simulink model "Body_Dynamics"  (R2020a)
settings: Solver=ode4  StartTime=0.0  StopTime=200  FixedStep=0.01  RelTol=1e-3
values from neighbouring files (symbols this model uses):
  A =     [bluntbody_parameters.m]
  alpha = [aero_data(19:-1:1,1);aero_data(20:38,1)]    [bluntbody_parameters.m]
  Cd = [aero_data(19:-1:1,3);aero_data(20:38,3)]    [bluntbody_parameters.m]
  Cl = [aero_data(19:-1:1,2);aero_data(20:38,2)]    [bluntbody_parameters.m]
  Cmalphadot =     [bluntbody_parameters.m]
  Cmcg = [aero_data(19:-1:1,9);aero_data(20:38,9)]    [bluntbody_parameters.m]
  Cmq =     [bluntbody_parameters.m]
  D =     [bluntbody_parameters.m]
  g =     [bluntbody_parameters.m]
  Iyy =     [bluntbody_parameters.m]
  Ka =     [bluntbody_parameters.m]
  Kr =     [bluntbody_parameters.m]
  lc =     [bluntbody_parameters.m]
  LTP =     [bluntbody_parameters.m]
  m =     [bluntbody_parameters.m]
  R =     [bluntbody_parameters.m]
  RCL =     [bluntbody_parameters.m]
  Tc =     [bluntbody_parameters.m]
  UTP =     [bluntbody_parameters.m]
settings Model: Creator=nikun  LastModifiedBy=nikun

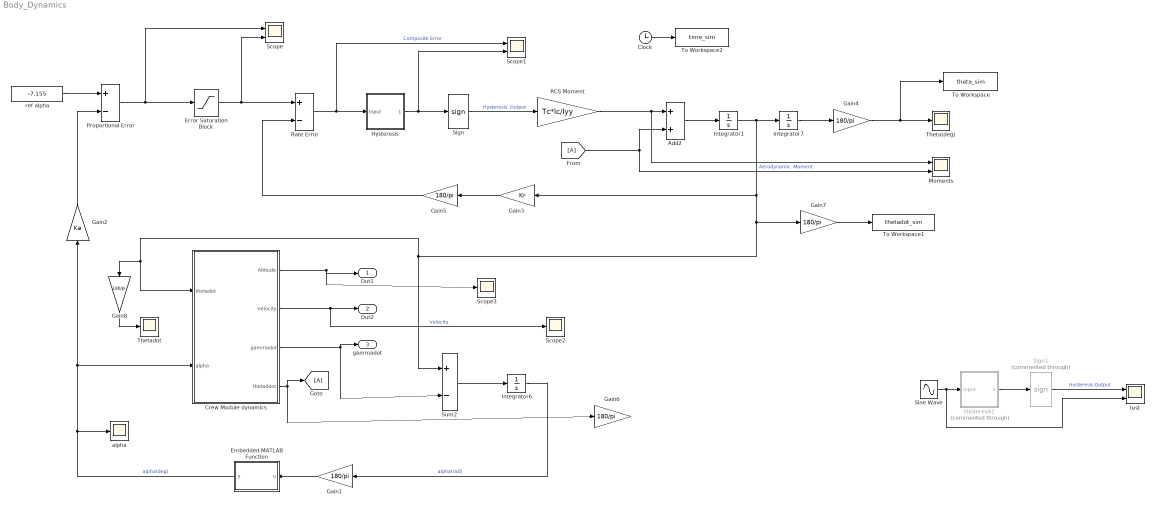
== system Body_Dynamics ==
  Add2 : Sum
  Clock : Clock
  Crew Module dynamics : Subsystem
  Embedded MATLAB Function : MATLAB Function  TreatAsAtomicUnit=on
  Error Saturation Block : Saturate  UpperLimit=RCL  LowerLimit=-RCL
  Gain{1,4..8} (6 alike) : Gain  Gain=180/pi  SaturateOnIntegerOverflow=on  OutDataTypeStr=Inherit: Same as input  ParamDataTypeStr=Inherit: Same as input
  Gain2 : Gain  Gain=Ka  SaturateOnIntegerOverflow=on  OutDataTypeStr=Inherit: Same as input  ParamDataTypeStr=Inherit: Same as input
  Gain3 : Gain  Gain=Kr  SaturateOnIntegerOverflow=on  OutDataTypeStr=Inherit: Same as input  ParamDataTypeStr=Inherit: Same as input
  Hysteresis : Subsystem
  Hysteresis1 : Subsystem  Commented=through
  Integrator1 : Integrator
  Integrator6 : Integrator  InitialCondition=150*pi/180
  Integrator7 : Integrator  InitialCondition=-2*pi/180
  Moments : Scope  NumInputPorts=2
  Proportional Error : Sum  Inputs=+-
  RCS Moment : Gain  Gain=Tc*lc/Iyy  SaturateOnIntegerOverflow=on  OutDataTypeStr=Inherit: Same as input  ParamDataTypeStr=Inherit: Same as input
  Rate Error : Sum  Inputs=+-
  Scope : Scope  NumInputPorts=2
  Scope1 : Scope  NumInputPorts=2
  Scope2 : Scope
  Scope3 : Scope
  Sign : Signum  ZeroCross=off
  Sign1 : Signum  Commented=through  ZeroCross=off
  Sine Wave : Sin  Amplitude=10  SampleTime=0
  Sum2 : Sum  Inputs=+-  InputSameDT=on  SaturateOnIntegerOverflow=on  OutDataTypeStr=Inherit: Same as first input
  Theta(deg) : Scope
  Thetadot : Scope
  To Workspace : ToWorkspace  VariableName=theta_sim  SampleTime=-1
  To Workspace1 : ToWorkspace  VariableName=thetadot_sim  SampleTime=-1
  To Workspace2 : ToWorkspace  VariableName=time_sim  SampleTime=-1
  alpha : Scope
  ref alpha : Constant  Value=-7.155
  test : Scope  NumInputPorts=2
  Out1 : Outport
  Out2 : Outport  Port=2
  gammadot : Outport  Port=3
  wires:
  Sum2/1 -> Integrator6/1
  Integrator6/1 -> Gain1/1  "alpha(rad)"
  Gain1/1 -> Embedded MATLAB Function/1(u)
  Crew Module dynamics/1(Altitude) -> Scope3/1, Out1/1
  Crew Module dynamics/2(Velocity) -> Scope2/1, Out2/1  "Velocity"
  Crew Module dynamics/3(gammadot) -> Sum2/2, gammadot/1
  Embedded MATLAB Function/1(y) -> alpha/1, Crew Module dynamics/2(alpha), Gain2/1  "alpha(deg)"
  Gain2/1 -> Proportional Error/2
  ref alpha/1 -> Proportional Error/1
  Proportional Error/1 -> Scope/1, Error Saturation Block/1
  Error Saturation Block/1 -> Scope/2, Rate Error/1
  Crew Module dynamics/4(thetaddot) -> Gain6/1, [A]
  [A] -> Moments/2, Add2/2  "Aerodynamic  Moment"
  Add2/1 -> Integrator1/1
  Integrator1/1 -> Gain3/1, Gain7/1, Gain8/1, Crew Module dynamics/1(thetadot), Sum2/1, Integrator7/1
  RCS Moment/1 -> Moments/1, Add2/1
  Sign/1 -> RCS Moment/1  "Hysteresis  Output"
  Gain3/1 -> Gain5/1
  Integrator7/1 -> Gain4/1
  Gain4/1 -> To Workspace/1, Theta(deg)/1
  Hysteresis/1(Output) -> Scope1/2, Sign/1
  Rate Error/1 -> Scope1/1, Hysteresis/1(Input)  "Composite Error"
  Gain5/1 -> Rate Error/2
  Sine Wave/1 -> test/2, Hysteresis1/1(Input)
  Hysteresis1/1(Output) -> Sign1/1
  Sign1/1 -> test/1  "Hysteresis Output"
  Gain7/1 -> To Workspace1/1
  Clock/1 -> To Workspace2/1
  Gain8/1 -> Thetadot/1

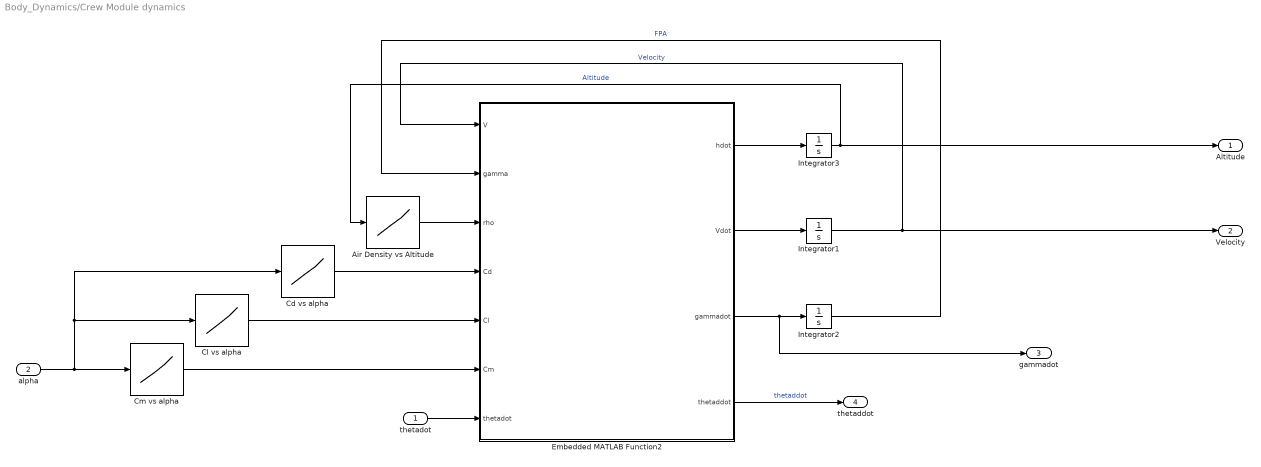
== system Body_Dynamics/Crew Module dynamics ==
  thetadot : Inport
  alpha : Inport  Port=2
  Air Density vs Altitude : Lookup_n-D  NumberOfTableDimensions=1  BreakpointsForDimension1=[0,1000,2000,3000,4000,5000,6000,7000,8000,9000,10000,12000,15000]  Table=[1.225,1.11164,1.00649,0.909122,0.819129,0.736116,0.659697,0.589501,0.525168,0.466348,0.412707,0.310828,0.193674]  InternalRulePriority=Speed  RndMeth=Simplest  InputSameDT=on
  Cd vs alpha : Lookup_n-D  NumberOfTableDimensions=1  BreakpointsForDimension1=alpha  Table=Cd  RndMeth=Simplest  InputSameDT=on
  Cl vs alpha : Lookup_n-D  NumberOfTableDimensions=1  BreakpointsForDimension1=alpha  Table=Cl  RndMeth=Simplest  InputSameDT=on
  Cm vs alpha : Lookup_n-D  NumberOfTableDimensions=1  BreakpointsForDimension1=alpha  Table=Cmcg  RndMeth=Simplest  InputSameDT=on
  Embedded MATLAB Function2 : MATLAB Function  TreatAsAtomicUnit=on
  Integrator1 : Integrator  InitialCondition=68
  Integrator2 : Integrator  InitialCondition=1*pi/180
  Integrator3 : Integrator  InitialCondition=13240
  Altitude : Outport
  Velocity : Outport  Port=2
  gammadot : Outport  Port=3
  thetaddot : Outport  Port=4
  wires:
  Embedded MATLAB Function2/4(thetaddot) -> thetaddot/1  "thetaddot"
  Embedded MATLAB Function2/2(Vdot) -> Integrator1/1
  Integrator2/1 -> Embedded MATLAB Function2/2(gamma)  "FPA"
  Integrator1/1 -> Velocity/1, Embedded MATLAB Function2/1(V)  "Velocity"
  Cl vs alpha/1 -> Embedded MATLAB Function2/5(Cl)
  alpha/1 -> Cd vs alpha/1, Cl vs alpha/1, Cm vs alpha/1
  Cd vs alpha/1 -> Embedded MATLAB Function2/4(Cd)
  Cm vs alpha/1 -> Embedded MATLAB Function2/6(Cm)
  Integrator3/1 -> Altitude/1, Air Density vs Altitude/1  "Altitude"
  Air Density vs Altitude/1 -> Embedded MATLAB Function2/3(rho)
  Embedded MATLAB Function2/1(hdot) -> Integrator3/1
  Embedded MATLAB Function2/3(gammadot) -> gammadot/1, Integrator2/1
  thetadot/1 -> Embedded MATLAB Function2/7(thetadot)

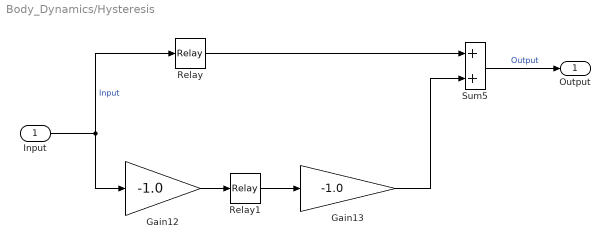
== system Body_Dynamics/Hysteresis ==
  Input : Inport
  Gain12 : Gain  Gain=-1.0  SaturateOnIntegerOverflow=on  OutDataTypeStr=Inherit: Same as input  ParamDataTypeStr=Inherit: Same as input
  Gain13 : Gain  Gain=-1.0  SaturateOnIntegerOverflow=on  OutDataTypeStr=Inherit: Same as input  ParamDataTypeStr=Inherit: Same as input
  Relay : Relay  OnSwitchValue=UTP  OffSwitchValue=LTP
  Relay1 : Relay  OnSwitchValue=UTP  OffSwitchValue=LTP
  Sum5 : Sum  InputSameDT=on  SaturateOnIntegerOverflow=on  OutDataTypeStr=Inherit: Same as first input
  Output : Outport
  wires:
  Relay/1 -> Sum5/1
  Input/1 -> Gain12/1, Relay/1  "Input"
  Sum5/1 -> Output/1  "Output"
  Gain12/1 -> Relay1/1
  Relay1/1 -> Gain13/1
  Gain13/1 -> Sum5/2

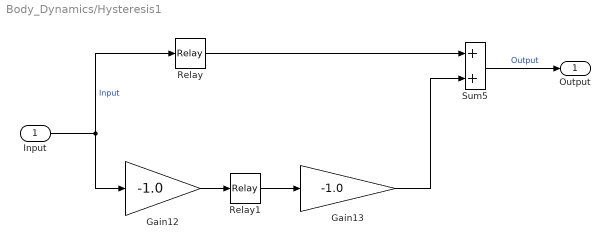
== system Body_Dynamics/Hysteresis1 ==
  Input : Inport
  Gain12 : Gain  Gain=-1.0  SaturateOnIntegerOverflow=on  OutDataTypeStr=Inherit: Same as input  ParamDataTypeStr=Inherit: Same as input
  Gain13 : Gain  Gain=-1.0  SaturateOnIntegerOverflow=on  OutDataTypeStr=Inherit: Same as input  ParamDataTypeStr=Inherit: Same as input
  Relay : Relay  OnSwitchValue=UTP  OffSwitchValue=LTP
  Relay1 : Relay  OnSwitchValue=UTP  OffSwitchValue=LTP
  Sum5 : Sum  InputSameDT=on  SaturateOnIntegerOverflow=on  OutDataTypeStr=Inherit: Same as first input
  Output : Outport
  wires:
  Relay/1 -> Sum5/1
  Input/1 -> Gain12/1, Relay/1  "Input"
  Sum5/1 -> Output/1  "Output"
  Gain12/1 -> Relay1/1
  Relay1/1 -> Gain13/1
  Gain13/1 -> Sum5/2

== matlab function Body_Dynamics/Embedded MATLAB Function ==
  data: u input; y output
function y = fcn(u)
%#eml
% if(u>0)
%     y = mod(u,360);
%     if(y > 180)
%        y = -180 + (y - 180);
%     end
%     
% else
%     y = -u;
%     y = -mod(y,360);
%     if(y<-180)
%         y = 180 - (-y + 180);
%     end
% end

x = mod(u,360);

if(x <= 180)
    y=x;
else
    y = x-360;
end
end

== matlab function Body_Dynamics/Crew Module dynamics/Embedded MATLAB Function2 ==
  data: V input; hdot output; gamma input; rho input; Cd input; A parameter; m parameter; g parameter; Cl input; R parameter; Iyy parameter; Cmq parameter; D parameter; Cmalphadot parameter; Cm input; thetadot input; Vdot output; gammadot output; thetaddot output
function [hdot, Vdot, gammadot, thetaddot] = fcn(V, gamma, rho, Cd, A, m, g,...
    Cl, R, Iyy, Cmq, D, Cmalphadot, Cm, thetadot)

hdot = V*sin(gamma);

Vdot = -(rho*V*V*Cd*A)/m - g*sin(gamma);
%  Vdot = 0;

gammadot = (rho*V*Cl*A)/(2*m) - (g/V - V/R)*cos(gamma);
% gammadot = 0;

thetaddot = ((rho*V*V*A*D)/(2*Iyy))*(((-Cmq-Cmalphadot)*thetadot*D)/(2*V) ...
     + Cm);                                                                         %%% Cmalpha*alpha = Cm
